simulink library "PIcontroller"  (R2017b)
settings: Solver=VariableStepAuto  StartTime=0.0  StopTime=10.0  RelTol=1e-3  EnableMultiTasking=on
undefined symbols (not defined in the file or in its folder): A, b, B, C, D, J, K, L, R
libraries: dspsigops x2
settings Model: Creator=qlong1505  LastModifiedBy=qlong1505
settings DataIOCC: LimitDataPoints=on
settings OptimizationCC: LifeSpan=inf
settings DebuggingCC: AllowSymbolicDim=off  SFUnexpectedBacktrackingDiag=warning  SFNoUnconditionalDefaultTransitionDiag=warning  SFExecutionAtInitializationDiag=none
settings ModelReferenceCC: PropagateSignalLabelsOutOfModel=off
settings CodeAppCC: StateflowObjectComments=on
settings GRTTargetCC: TargetLangStandard=C89/C90 (ANSI)
settings ConfigComp: CovMetricSettings=dw  CovHtmlReporting=on  CovSaveCumulativeToWorkspaceVar=on  CovSaveSingleToWorkspaceVar=on  CovExternalEMLEnable=off

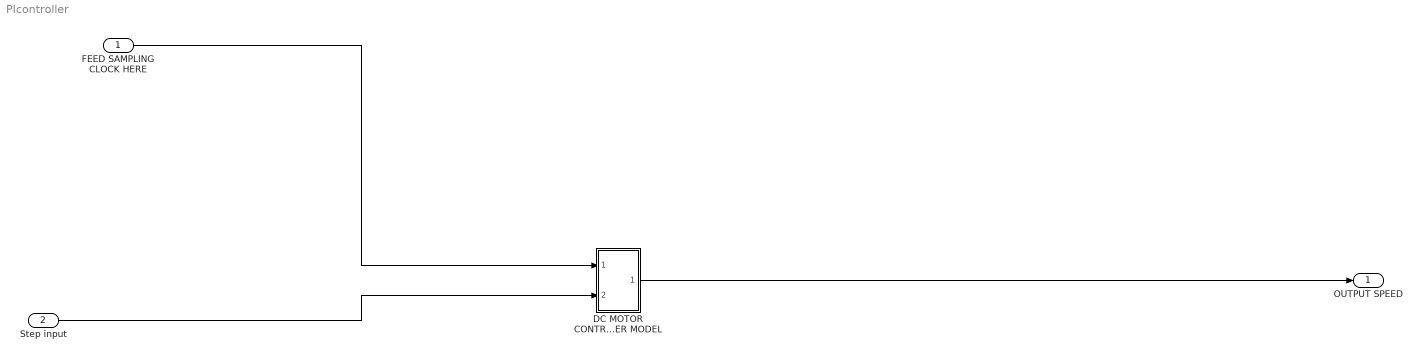
== system PIcontroller ==
  FEED SAMPLING CLOCK HERE : Inport
  Step input : Inport  Port=2
  DC MOTOR CONTROLLER MODEL : Subsystem
  OUTPUT SPEED : Outport
  wires:
  FEED SAMPLING CLOCK HERE/1 -> DC MOTOR CONTROLLER MODEL/1(FEED SAMPLING CLOCK HERE)
  Step input/1 -> DC MOTOR CONTROLLER MODEL/2(Step input)
  DC MOTOR CONTROLLER MODEL/1(OUTPUT SPEED) -> OUTPUT SPEED/1

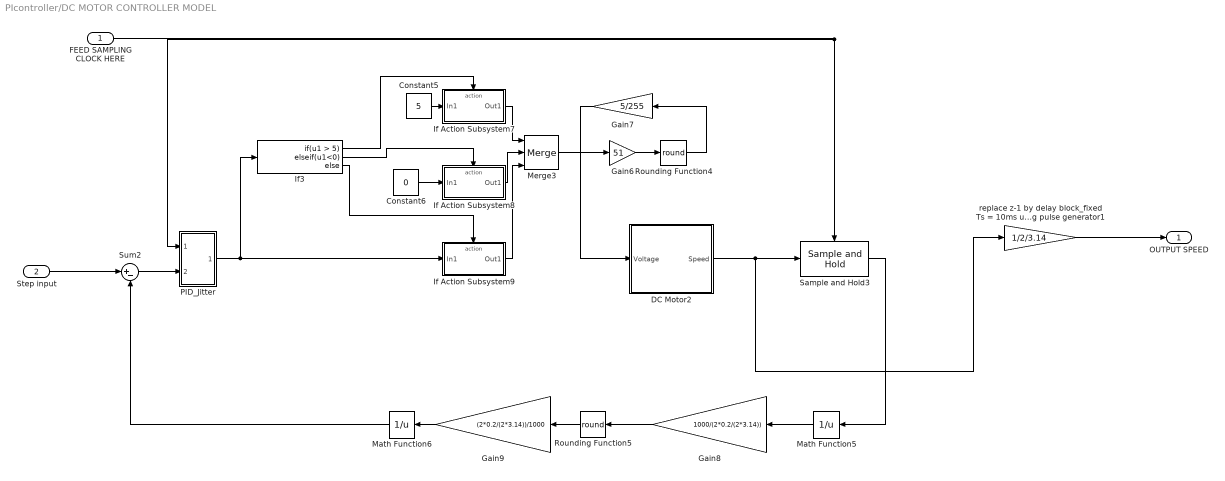
== system PIcontroller/DC MOTOR CONTROLLER MODEL ==
  FEED SAMPLING CLOCK HERE : Inport
  Step input : Inport  Port=2
  Constant5 : Constant  Value=5
  Constant6 : Constant  Value=0
  DC Motor2 : Subsystem
  Gain6 : Gain  Gain=51
  Gain7 : Gain  Gain=5/255
  Gain8 : Gain  Gain=1000/(2*0.2/(2*3.14))
  Gain9 : Gain  Gain=(2*0.2/(2*3.14))/1000
  If Action Subsystem7 : Subsystem  TreatAsAtomicUnit=on
  If Action Subsystem8 : Subsystem  TreatAsAtomicUnit=on
  If Action Subsystem9 : Subsystem  TreatAsAtomicUnit=on
  If3 : If  IfExpression=u1 > 5  ElseIfExpressions=u1<0
  Math Function5 : Math  Operator=reciprocal  SaturateOnIntegerOverflow=on
  Math Function6 : Math  Operator=reciprocal  SaturateOnIntegerOverflow=on
  Merge3 : Merge  Inputs=3
  PID_Jitter : Subsystem
  Rounding Function4 : Rounding  Operator=round
  Rounding Function5 : Rounding  Operator=round
  Sample and Hold3 : dspsigops/Sample and Hold  trig=Rising edge  initCond=0  latchinput=on
  Sum2 : Sum  Inputs=|+-
  replace z-1 by delay block_fixed Ts = 10ms using pulse generator1 : Gain  Gain=1/2/3.14
  OUTPUT SPEED : Outport
  wires:
  Rounding Function5/1 -> Gain9/1
  Math Function6/1 -> Sum2/2
  Constant5/1 -> If Action Subsystem7/1(In1)
  If3/2 -> If Action Subsystem8/Action
  replace z-1 by delay block_fixed Ts = 10ms using pulse generator1/1 -> OUTPUT SPEED/1
  Sum2/1 -> PID_Jitter/2(In2)
  Sample and Hold3/1 -> Math Function5/1
  Gain8/1 -> Rounding Function5/1
  FEED SAMPLING CLOCK HERE/1 -> Sample and Hold3/Trigger, PID_Jitter/1(clock jitter)
  Merge3/1 -> Gain6/1
  If Action Subsystem7/1(Out1) -> Merge3/1
  If3/1 -> If Action Subsystem7/Action
  Constant6/1 -> If Action Subsystem8/1(In1)
  DC Motor2/1(" Speed") -> Sample and Hold3/1, replace z-1 by delay block_fixed Ts = 10ms using pulse generator1/1
  Rounding Function4/1 -> Gain7/1
  PID_Jitter/1(Out1) -> If3/1, If Action Subsystem9/1(In1)
  If3/3 -> If Action Subsystem9/Action
  Gain9/1 -> Math Function6/1
  Math Function5/1 -> Gain8/1
  Gain6/1 -> Rounding Function4/1
  If Action Subsystem9/1(Out1) -> Merge3/3
  Gain7/1 -> DC Motor2/1(Voltage)
  If Action Subsystem8/1(Out1) -> Merge3/2
  Step input/1 -> Sum2/1

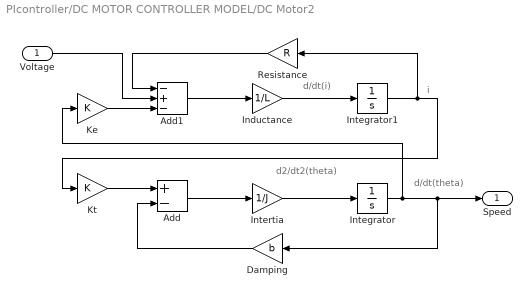
== system PIcontroller/DC MOTOR CONTROLLER MODEL/DC Motor2 ==
  note: i
  note: d/dt(theta)
  note: d2/dt2(theta)
  note: d/dt(i)
  Voltage : Inport
  Add : Sum  Inputs=+-
  Add1 : Sum  Inputs=-+-
  Damping : Gain  Gain=b
  Inductance : Gain  Gain=1/L
  Integrator : Integrator
  Integrator1 : Integrator
  Intertia : Gain  Gain=1/J
  Ke : Gain  Gain=K
  Kt : Gain  Gain=K
  Resistance : Gain  Gain=R
  " Speed" : Outport
  wires:
  Integrator1/1 -> Kt/1, Resistance/1
  Inductance/1 -> Integrator1/1
  Intertia/1 -> Integrator/1
  Integrator/1 -> Ke/1, Damping/1, " Speed"/1
  Add1/1 -> Inductance/1
  Add/1 -> Intertia/1
  Damping/1 -> Add/2
  Kt/1 -> Add/1
  Resistance/1 -> Add1/1
  Ke/1 -> Add1/3
  Voltage/1 -> Add1/2

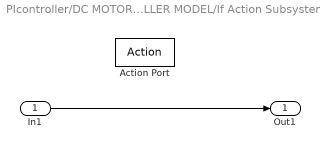
== system PIcontroller/DC MOTOR CONTROLLER MODEL/If Action Subsystem7 ==
  In1 : Inport
  Action Port : ActionPort
  Out1 : Outport
  wires:
  In1/1 -> Out1/1

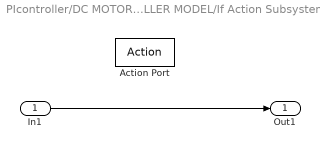
== system PIcontroller/DC MOTOR CONTROLLER MODEL/If Action Subsystem8 ==
  In1 : Inport
  Action Port : ActionPort
  Out1 : Outport
  wires:
  In1/1 -> Out1/1

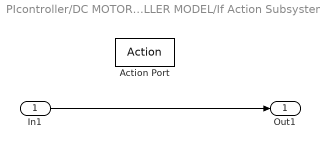
== system PIcontroller/DC MOTOR CONTROLLER MODEL/If Action Subsystem9 ==
  In1 : Inport
  Action Port : ActionPort
  Out1 : Outport
  wires:
  In1/1 -> Out1/1

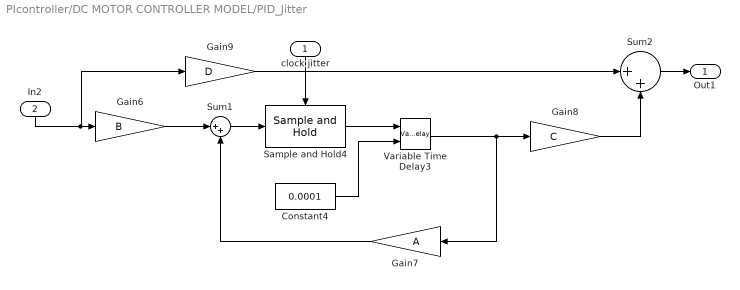
== system PIcontroller/DC MOTOR CONTROLLER MODEL/PID_Jitter ==
  clock jitter : Inport
  In2 : Inport  Port=2
  Constant4 : Constant  Value=0.0001  SampleTime=0.01
  Gain6 : Gain  Gain=B
  Gain7 : Gain  Gain=A
  Gain8 : Gain  Gain=C
  Gain9 : Gain  Gain=D
  Sample and Hold4 : dspsigops/Sample and Hold  trig=Rising edge  initCond=0  latchinput=on
  Sum1 : Sum  Inputs=|++
  Sum2 : Sum  Inputs=|++
  Variable Time Delay3 : VariableTransportDelay  VariableDelayType=Variable transport delay  MaximumDelay=10
  Out1 : Outport
  wires:
  Sample and Hold4/1 -> Variable Time Delay3/1
  Gain8/1 -> Sum2/2
  Variable Time Delay3/1 -> Gain8/1, Gain7/1
  Gain6/1 -> Sum1/1
  Sum1/1 -> Sample and Hold4/1
  Gain7/1 -> Sum1/2
  Gain9/1 -> Sum2/1
  Constant4/1 -> Variable Time Delay3/2
  clock jitter/1 -> Sample and Hold4/Trigger
  Sum2/1 -> Out1/1
  In2/1 -> Gain9/1, Gain6/1
